simulink model "fp_demo"  (Simulink 6.3)
settings: Solver=FixedStepDiscrete  StartTime=0.0  StopTime=samps+8  RelTol=1e-3
PreLoadFcn:
  | testmult
InitFcn:
  | %% DSPBuilder Start
  | alt_dspbuilder_update_model(bdroot)
  | %% DSPBuilder End
undefined symbols (not defined in the file or in its folder): fplib, FPMULT_HW
libraries: allblocks_alteradspbuilder2 x112
settings Model: Creator=mjervis  LastModifiedBy=LKONG
settings OptimizationCC: InlineInvariantSignals=on
settings DebuggingCC: SolverPrmCheckMsg=none
settings HardwareCC: TargetUnknown=on

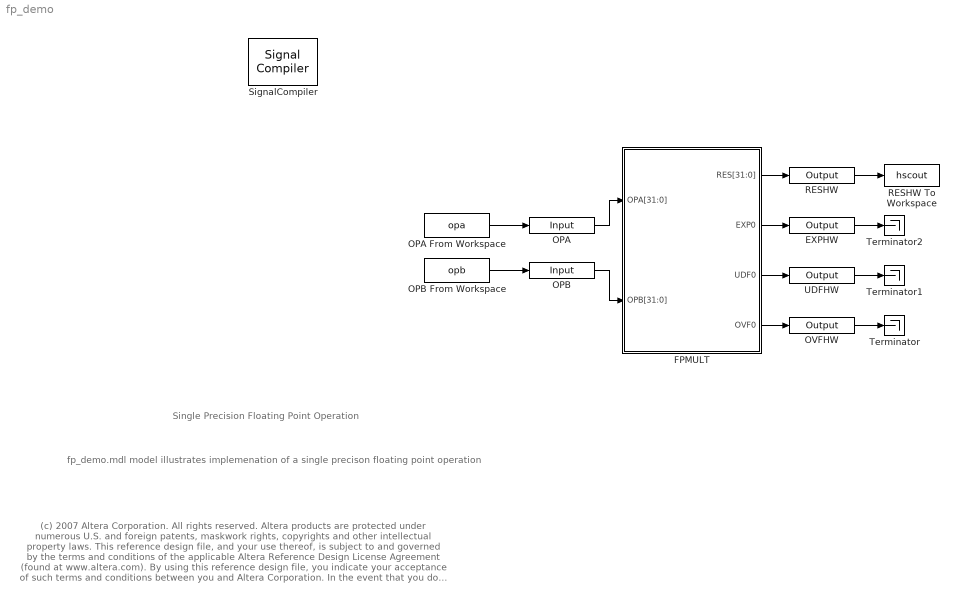
== system fp_demo ==
  note: (c) 2007 Altera Corporation. All rights reserved.  Altera products are protected under numerous U.S. and foreign patents, maskwork rights, copyrights and other intellectual property laws.
      | This reference design file, and your use thereof, is subject to and governed by the terms and conditions of the applicable Altera Reference Design License Agreement (found at www.altera.com).
      | By using this reference design file, you indicate your acceptance of such terms and conditions between you and Altera Corporation.
      | In the event that you do not agree with such terms and conditions, you may not use the reference design file and please promptly destroy any copies you have made.
      | This reference design file being provided on an "as-is" basis and as an accommodation and therefore all warranties, representations or guarantees of any kind (whether express, implied or statutory)
      | including, without limitation, warranties of merchantability, non-infringement, or fitness for a particular purpose, are specifically disclaimed.
      | By making this reference design file available, Altera expressly does not recommend, suggest or require that this reference design file be used in combination with any other product not provided by Altera
  note: Single Precision Floating Point Operation
  note: fp_demo.mdl model illustrates implemenation of a single precison floating point operation
  EXPHW : allblocks_alteradspbuilder2/Output  iofile=d:\wsTrunk\workspace\Documentation\DesignExamples\Demos\fp\Arithm\tb_fp_demo\fp_demo_EXPHW.capture  BusType=Single Bit  bwl=1  bwr=0  PORTTYPE=Output
  FPMULT : Subsystem  AncestorBlock=fplib/FPMULT_HW
      mask Type: SubSystem AlteraBlockSet
  OPA : allblocks_alteradspbuilder2/Input  iofile=d:\wsTrunk\workspace\Documentation\DesignExamples\Demos\fp\Arithm\tb_fp_demo\fp_demo_OPA.salt  BusType=Unsigned Integer  bwl=32  bwr=0  SpecifyClock=off  PORTTYPE=Input
  OPA From Workspace : FromWorkspace  VariableName=opa  SampleTime=1  Interpolate=off  OutputAfterFinalValue=Setting to zero
  OPB : allblocks_alteradspbuilder2/Input  iofile=d:\wsTrunk\workspace\Documentation\DesignExamples\Demos\fp\Arithm\tb_fp_demo\fp_demo_OPB.salt  BusType=Unsigned Integer  bwl=32  bwr=0  SpecifyClock=off  PORTTYPE=Input
  OPB From Workspace : FromWorkspace  VariableName=opb  SampleTime=1  Interpolate=off  OutputAfterFinalValue=Setting to zero
  OVFHW : allblocks_alteradspbuilder2/Output  iofile=d:\wsTrunk\workspace\Documentation\DesignExamples\Demos\fp\Arithm\tb_fp_demo\fp_demo_OVFHW.capture  BusType=Single Bit  bwl=1  bwr=0  PORTTYPE=Output
  RESHW : allblocks_alteradspbuilder2/Output  iofile=d:\wsTrunk\workspace\Documentation\DesignExamples\Demos\fp\Arithm\tb_fp_demo\fp_demo_RESHW.capture  BusType=Unsigned Integer  bwl=32  bwr=0  PORTTYPE=Output
  RESHW To Workspace : ToWorkspace  VariableName=hscout  SampleTime=-1  SaveFormat=Array
  SignalCompiler : allblocks_alteradspbuilder2/Signal Compiler  DeviceFamily=Stratix III  DeviceName=AUTO  EnableSignalTap=off  SignalTapDepth=128  UseBoardBlock=off  StpUseDefaultClock=on  StpClock=clock
  Terminator : Terminator
  Terminator1 : Terminator
  Terminator2 : Terminator
  UDFHW : allblocks_alteradspbuilder2/Output  iofile=d:\wsTrunk\workspace\Documentation\DesignExamples\Demos\fp\Arithm\tb_fp_demo\fp_demo_UDFHW.capture  BusType=Single Bit  bwl=1  bwr=0  PORTTYPE=Output
  wires:
  FPMULT/1(RES[31:0]) -> RESHW/1
  FPMULT/2(EXP0) -> EXPHW/1
  FPMULT/3(UDF0) -> UDFHW/1
  FPMULT/4(OVF0) -> OVFHW/1
  RESHW/1 -> RESHW To Workspace/1
  OPA From Workspace/1 -> OPA/1
  OPB From Workspace/1 -> OPB/1
  OPB/1 -> FPMULT/2(OPB[31:0])
  OPA/1 -> FPMULT/1(OPA[31:0])
  OVFHW/1 -> Terminator/1
  EXPHW/1 -> Terminator2/1
  UDFHW/1 -> Terminator1/1

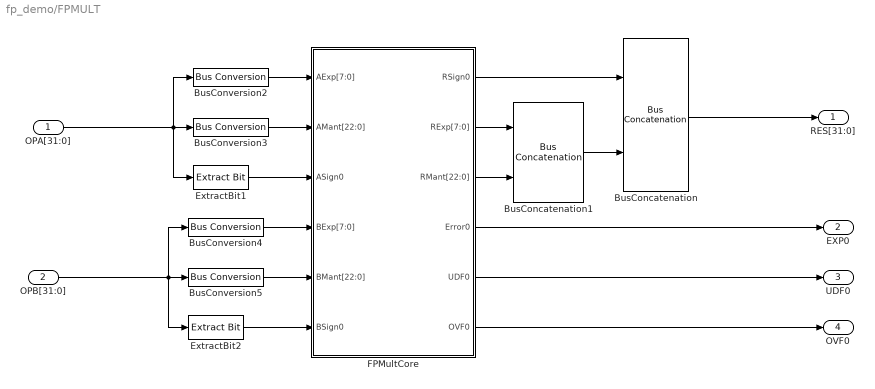
== system fp_demo/FPMULT ==
  OPA[31:0] : Inport
  OPB[31:0] : Inport  Port=2
  BusConcatenation : allblocks_alteradspbuilder2/Bus Concatenation  isSigned=off  awidth=1  bwidth=31
  BusConcatenation1 : allblocks_alteradspbuilder2/Bus Concatenation  isSigned=off  awidth=8  bwidth=23
  BusConversion2 : allblocks_alteradspbuilder2/Bus Conversion  BusType=Unsigned Integer  ibwl=32  ibwr=0  bwl=8  bwr=0  bitToConnectToOutputLSB=23  round=off  saturate=off
  BusConversion3 : allblocks_alteradspbuilder2/Bus Conversion  BusType=Unsigned Integer  ibwl=32  ibwr=0  bwl=23  bwr=0  bitToConnectToOutputLSB=0  round=off  saturate=off
  BusConversion4 : allblocks_alteradspbuilder2/Bus Conversion  BusType=Unsigned Integer  ibwl=32  ibwr=0  bwl=8  bwr=0  bitToConnectToOutputLSB=23  round=off  saturate=off
  BusConversion5 : allblocks_alteradspbuilder2/Bus Conversion  BusType=Unsigned Integer  ibwl=32  ibwr=0  bwl=23  bwr=0  bitToConnectToOutputLSB=0  round=off  saturate=off
  ExtractBit1 : allblocks_alteradspbuilder2/Extract Bit  BusType=Signed Fractional  bwl=32  bwr=0  bitToSelect=31
  ExtractBit2 : allblocks_alteradspbuilder2/Extract Bit  BusType=Signed Fractional  bwl=32  bwr=0  bitToSelect=31
  FPMultCore : Subsystem  AncestorBlock=ALTELINK/AltLab/HDL SubSystem
      mask Type: SubSystem AlteraBlockSet
  RES[31:0] : Outport
  EXP0 : Outport  Port=2
  UDF0 : Outport  Port=3
  OVF0 : Outport  Port=4
  wires:
  FPMultCore/6(OVF0) -> OVF0/1
  FPMultCore/5(UDF0) -> UDF0/1
  FPMultCore/4(Error0) -> EXP0/1
  BusConcatenation/1 -> RES[31:0]/1
  BusConcatenation1/1 -> BusConcatenation/2
  FPMultCore/2(RExp[7:0]) -> BusConcatenation1/1
  FPMultCore/3(RMant[22:0]) -> BusConcatenation1/2
  FPMultCore/1(RSign0) -> BusConcatenation/1
  ExtractBit2/1 -> FPMultCore/6(BSign0)
  BusConversion5/1 -> FPMultCore/5(BMant[22:0])
  BusConversion4/1 -> FPMultCore/4(BExp[7:0])
  ExtractBit1/1 -> FPMultCore/3(ASign0)
  BusConversion3/1 -> FPMultCore/2(AMant[22:0])
  BusConversion2/1 -> FPMultCore/1(AExp[7:0])
  OPA[31:0]/1 -> ExtractBit1/1, BusConversion3/1, BusConversion2/1
  OPB[31:0]/1 -> BusConversion4/1, BusConversion5/1, ExtractBit2/1

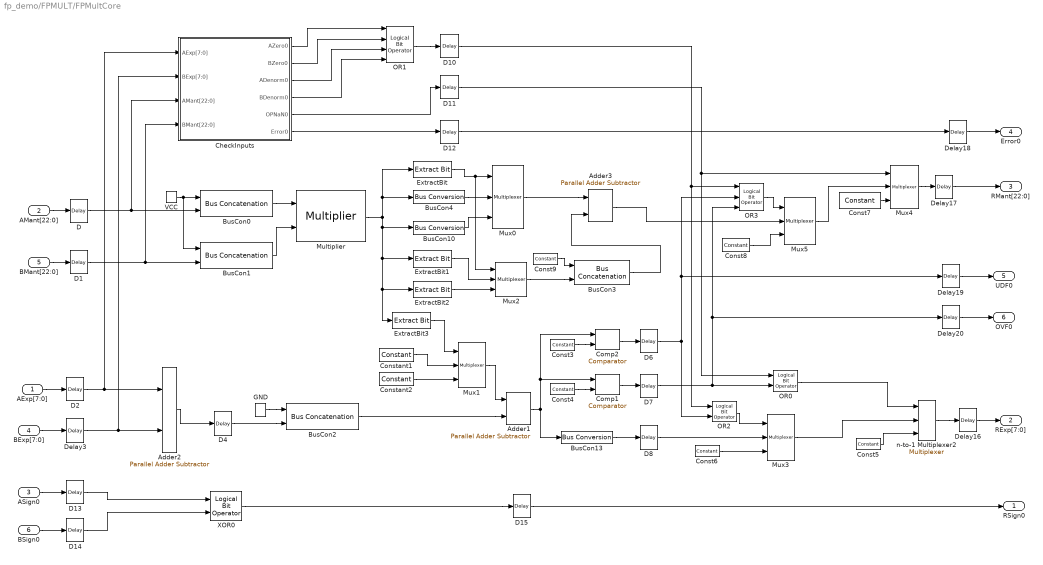
== system fp_demo/FPMULT/FPMultCore ==
  AExp[7:0] : Inport
  AMant[22:0] : Inport  Port=2
  ASign0 : Inport  Port=3
  BExp[7:0] : Inport  Port=4
  BMant[22:0] : Inport  Port=5
  BSign0 : Inport  Port=6
  Adder1 : allblocks_alteradspbuilder2/Parallel Adder Subtractor  number_of_inputs=2  direction=-+  use_pipeline=on  phase_selection=1  use_ena=off  use_aclr=off
  Adder2 : allblocks_alteradspbuilder2/Parallel Adder Subtractor  number_of_inputs=2  direction=++  use_pipeline=on  phase_selection=1  use_ena=off  use_aclr=off
  Adder3 : allblocks_alteradspbuilder2/Parallel Adder Subtractor  number_of_inputs=2  direction=++  use_pipeline=on  phase_selection=1  use_ena=off  use_aclr=off
  BusCon0 : allblocks_alteradspbuilder2/Bus Concatenation  isSigned=off  awidth=1  bwidth=23
  BusCon1 : allblocks_alteradspbuilder2/Bus Concatenation  isSigned=off  awidth=1  bwidth=23
  BusCon10 : allblocks_alteradspbuilder2/Bus Conversion  BusType=Unsigned Integer  ibwl=48  ibwr=0  bwl=23  bwr=0  bitToConnectToOutputLSB=24  round=off  saturate=off
  BusCon13 : allblocks_alteradspbuilder2/Bus Conversion  BusType=Unsigned Integer  ibwl=11  ibwr=0  bwl=8  bwr=0  bitToConnectToOutputLSB=0  round=on  saturate=on
  BusCon2 : allblocks_alteradspbuilder2/Bus Concatenation  isSigned=on  awidth=1  bwidth=9
  BusCon3 : allblocks_alteradspbuilder2/Bus Concatenation  isSigned=off  awidth=22  bwidth=1
  BusCon4 : allblocks_alteradspbuilder2/Bus Conversion  BusType=Unsigned Integer  ibwl=48  ibwr=0  bwl=23  bwr=0  bitToConnectToOutputLSB=23  round=off  saturate=off
  CheckInputs : Subsystem  AncestorBlock=ALTELINK/AltLab/HDL SubSystem
      mask Type: SubSystem AlteraBlockSet
  Comp1 : allblocks_alteradspbuilder2/Comparator  direction=a >= b
  Comp2 : allblocks_alteradspbuilder2/Comparator  direction=a <= b
  Const3 : allblocks_alteradspbuilder2/Constant  mask_cst=0  BusType=Signed Integer  bwl=11  bwr=0  SpecifyClock=off
  Const4 : allblocks_alteradspbuilder2/Constant  mask_cst=255  BusType=Signed Integer  bwl=11  bwr=0  SpecifyClock=off
  Const5 : allblocks_alteradspbuilder2/Constant  mask_cst=255  BusType=Unsigned Integer  bwl=8  bwr=0  SpecifyClock=off
  Const6 : allblocks_alteradspbuilder2/Constant  mask_cst=0  BusType=Unsigned Integer  bwl=8  bwr=0  SpecifyClock=off
  Const7 : allblocks_alteradspbuilder2/Constant  mask_cst=(2^23)-1  BusType=Unsigned Integer  bwl=23  bwr=0  SpecifyClock=off
  Const8 : allblocks_alteradspbuilder2/Constant  mask_cst=0  BusType=Unsigned Integer  bwl=23  bwr=0  SpecifyClock=off
  Const9 : allblocks_alteradspbuilder2/Constant  mask_cst=0  BusType=Unsigned Integer  bwl=22  bwr=0  SpecifyClock=off
  Constant1 : allblocks_alteradspbuilder2/Constant  mask_cst=127  BusType=Signed Integer  bwl=10  bwr=0  SpecifyClock=off
  Constant2 : allblocks_alteradspbuilder2/Constant  mask_cst=126  BusType=Signed Integer  bwl=10  bwr=0  SpecifyClock=off
  D{,1..2,6..8,13..14} (8 alike) : allblocks_alteradspbuilder2/Delay  pipeline=1  ClockPhase=1  use_ena=off  use_sclr=off  use_init=off  reset_value=1
  D10 : allblocks_alteradspbuilder2/Delay  pipeline=4  ClockPhase=1  use_ena=off  use_sclr=off  use_init=off  reset_value=1
  D11 : allblocks_alteradspbuilder2/Delay  pipeline=4  ClockPhase=1  use_ena=off  use_sclr=off  use_init=off  reset_value=1
  D12 : allblocks_alteradspbuilder2/Delay  pipeline=5  ClockPhase=1  use_ena=off  use_sclr=off  use_init=off  reset_value=1
  D15 : allblocks_alteradspbuilder2/Delay  pipeline=6  ClockPhase=1  use_ena=off  use_sclr=off  use_init=off  reset_value=1
  D4 : allblocks_alteradspbuilder2/Delay  pipeline=2  ClockPhase=1  use_ena=off  use_sclr=off  use_init=off  reset_value=1
  Delay{3,16..20} (6 alike) : allblocks_alteradspbuilder2/Delay  pipeline=1  ClockPhase=1  use_ena=off  use_sclr=off  use_init=off  reset_value=1
  ExtractBit : allblocks_alteradspbuilder2/Extract Bit  BusType=Signed Fractional  bwl=48  bwr=0  bitToSelect=47
  ExtractBit1 : allblocks_alteradspbuilder2/Extract Bit  BusType=Signed Fractional  bwl=48  bwr=0  bitToSelect=22
  ExtractBit2 : allblocks_alteradspbuilder2/Extract Bit  BusType=Signed Fractional  bwl=48  bwr=0  bitToSelect=23
  ExtractBit3 : allblocks_alteradspbuilder2/Extract Bit  BusType=Signed Fractional  bwl=48  bwr=0  bitToSelect=47
  GND : allblocks_alteradspbuilder2/GND  SpecifyClock=off
  Multiplier : allblocks_alteradspbuilder2/Multiplier  BusType=Unsigned Integer  bwl=24  bwr=0  pipeline=3  UseEqualInputWidth=on  bbwl=24  bbwr=0  FullResolution=on  OutputMsb=47  OutputLsb=0  OutputBwl=48  OutputBwr=0  UseDedicatedCircuitry=AUTO  use_ena=off  use_aclr=off
  Mux0 : allblocks_alteradspbuilder2/Multiplexer  numInputs=2  pipeline=1  oneHot=off  use_ena=off  use_aclr=off
  Mux{1,3..5} (4 alike) : allblocks_alteradspbuilder2/Multiplexer  numInputs=2  pipeline=0  oneHot=off  use_ena=off  use_aclr=off
  Mux2 : allblocks_alteradspbuilder2/Multiplexer  numInputs=2  pipeline=1  oneHot=off  use_ena=off  use_aclr=off
  OR0 : allblocks_alteradspbuilder2/Logical Bit Operator  LogicalOperator=OR  user_inputs=2
  OR1 : allblocks_alteradspbuilder2/Logical Bit Operator  LogicalOperator=OR  user_inputs=4
  OR2 : allblocks_alteradspbuilder2/Logical Bit Operator  LogicalOperator=OR  user_inputs=2
  OR3 : allblocks_alteradspbuilder2/Logical Bit Operator  LogicalOperator=OR  user_inputs=3
  VCC : allblocks_alteradspbuilder2/VCC  SpecifyClock=off
  XOR0 : allblocks_alteradspbuilder2/Logical Bit Operator  LogicalOperator=XOR  user_inputs=2
  n-to-1 Multiplexer2 : allblocks_alteradspbuilder2/Multiplexer  numInputs=2  pipeline=0  oneHot=off  use_ena=off  use_aclr=off
  RSign0 : Outport
  RExp[7:0] : Outport  Port=2
  RMant[22:0] : Outport  Port=3
  Error0 : Outport  Port=4
  UDF0 : Outport  Port=5
  OVF0 : Outport  Port=6
  wires:
  Const8/1 -> Mux5/3
  OR3/1 -> Mux5/1
  CheckInputs/1(AZero0) -> OR1/1
  ExtractBit3/1 -> Mux1/1
  D2/1 -> CheckInputs/1(AExp[7:0]), Adder2/1
  Delay3/1 -> CheckInputs/2(BExp[7:0]), Adder2/2
  Const9/1 -> BusCon3/1
  Mux2/1 -> BusCon3/2
  BusCon3/1 -> Adder3/2
  ExtractBit1/1 -> Mux2/2
  ExtractBit2/1 -> Mux2/3
  Adder3/1 -> Mux5/2
  Mux0/1 -> Adder3/1
  Delay20/1 -> OVF0/1
  Delay19/1 -> UDF0/1
  Delay18/1 -> Error0/1
  D12/1 -> Delay18/1
  Delay17/1 -> RMant[22:0]/1
  Delay16/1 -> RExp[7:0]/1
  Mux4/1 -> Delay17/1
  n-to-1 Multiplexer2/1 -> Delay16/1
  XOR0/1 -> D15/1
  D14/1 -> XOR0/2
  D13/1 -> XOR0/1
  BSign0/1 -> D14/1
  ASign0/1 -> D13/1
  Mux5/1 -> Mux4/2
  Const7/1 -> Mux4/3
  D10/1 -> OR3/1, OR2/1
  D8/1 -> Mux3/2
  D6/1 -> OR2/2, OR3/2, Delay19/1
  OR2/1 -> Mux3/1
  Const6/1 -> Mux3/3
  Mux3/1 -> n-to-1 Multiplexer2/2
  Const5/1 -> n-to-1 Multiplexer2/3
  D11/1 -> OR0/1, Mux4/1
  D7/1 -> Delay20/1, OR3/3, OR0/2
  OR1/1 -> D10/1
  OR0/1 -> n-to-1 Multiplexer2/1
  CheckInputs/6(Error0) -> D12/1
  CheckInputs/5(OPNaN0) -> D11/1
  CheckInputs/4(BDenorm0) -> OR1/4
  CheckInputs/3(ADenorm0) -> OR1/3
  CheckInputs/2(BZero0) -> OR1/2
  BusCon13/1 -> D8/1
  Comp1/1 -> D7/1
  Comp2/1 -> D6/1
  Const4/1 -> Comp1/2
  Const3/1 -> Comp2/2
  Adder1/1 -> Comp1/1, Comp2/1, BusCon13/1
  GND/1 -> BusCon2/1
  BusCon2/1 -> Adder1/2
  Mux1/1 -> Adder1/1
  Constant2/1 -> Mux1/3
  Constant1/1 -> Mux1/2
  D4/1 -> BusCon2/2
  Adder2/1 -> D4/1
  ExtractBit/1 -> Mux2/1, Mux0/1
  BusCon10/1 -> Mux0/3
  BusCon4/1 -> Mux0/2
  VCC/1 -> BusCon0/1, BusCon1/1
  BusCon1/1 -> Multiplier/2
  BusCon0/1 -> Multiplier/1
  BMant[22:0]/1 -> D1/1
  BExp[7:0]/1 -> Delay3/1
  AMant[22:0]/1 -> D/1
  AExp[7:0]/1 -> D2/1
  D/1 -> BusCon0/2, CheckInputs/3(AMant[22:0])
  D1/1 -> BusCon1/2, CheckInputs/4(BMant[22:0])
  Multiplier/1 -> ExtractBit/1, BusCon4/1, BusCon10/1, ExtractBit1/1, ExtractBit3/1, ExtractBit2/1
  D15/1 -> RSign0/1

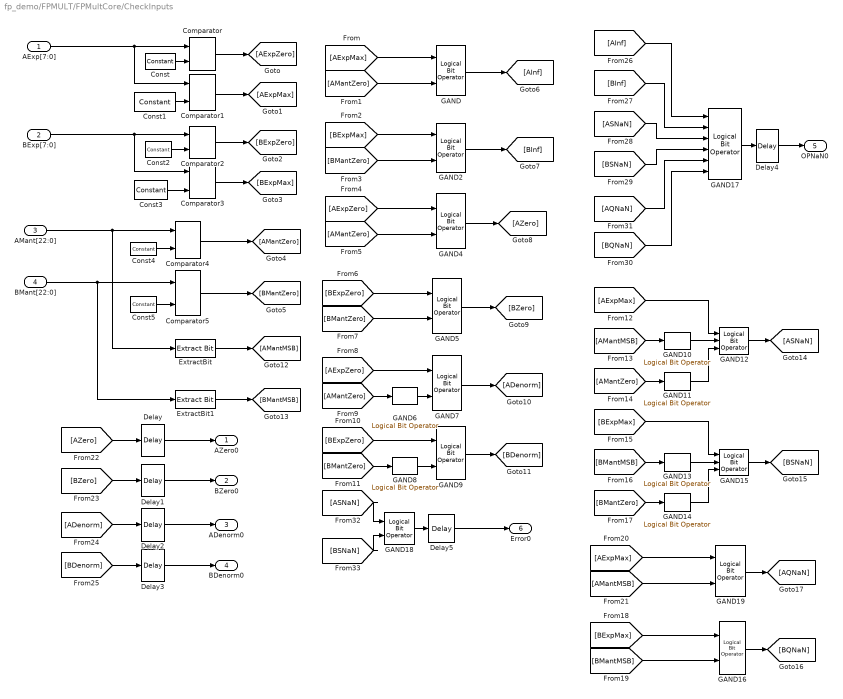
== system fp_demo/FPMULT/FPMultCore/CheckInputs ==
  AExp[7:0] : Inport
  BExp[7:0] : Inport  Port=2
  AMant[22:0] : Inport  Port=3
  BMant[22:0] : Inport  Port=4
  Comparator{,1..5} (6 alike) : allblocks_alteradspbuilder2/Comparator  direction=a == b
  Const : allblocks_alteradspbuilder2/Constant  mask_cst=0  BusType=Unsigned Integer  bwl=8  bwr=0  SpecifyClock=off
  Const1 : allblocks_alteradspbuilder2/Constant  mask_cst=255  BusType=Unsigned Integer  bwl=8  bwr=0  SpecifyClock=off
  Const2 : allblocks_alteradspbuilder2/Constant  mask_cst=0  BusType=Unsigned Integer  bwl=8  bwr=0  SpecifyClock=off
  Const3 : allblocks_alteradspbuilder2/Constant  mask_cst=255  BusType=Unsigned Integer  bwl=8  bwr=0  SpecifyClock=off
  Const4 : allblocks_alteradspbuilder2/Constant  mask_cst=0  BusType=Unsigned Integer  bwl=23  bwr=0  SpecifyClock=off
  Const5 : allblocks_alteradspbuilder2/Constant  mask_cst=0  BusType=Unsigned Integer  bwl=23  bwr=0  SpecifyClock=off
  Delay{,1..5} (6 alike) : allblocks_alteradspbuilder2/Delay  pipeline=1  ClockPhase=1  use_ena=off  use_sclr=off  use_init=off  reset_value=1
  ExtractBit : allblocks_alteradspbuilder2/Extract Bit  BusType=Signed Fractional  bwl=23  bwr=0  bitToSelect=22
  ExtractBit1 : allblocks_alteradspbuilder2/Extract Bit  BusType=Signed Fractional  bwl=23  bwr=0  bitToSelect=22
  GAND{,2,4..5,7,9,16,19} (8 alike) : allblocks_alteradspbuilder2/Logical Bit Operator  LogicalOperator=AND  user_inputs=2
  GAND{6,8,10..11,13..14} (6 alike) : allblocks_alteradspbuilder2/Logical Bit Operator  LogicalOperator=NOT  user_inputs=2
  GAND12 : allblocks_alteradspbuilder2/Logical Bit Operator  LogicalOperator=AND  user_inputs=3
  GAND15 : allblocks_alteradspbuilder2/Logical Bit Operator  LogicalOperator=AND  user_inputs=3
  GAND17 : allblocks_alteradspbuilder2/Logical Bit Operator  LogicalOperator=OR  user_inputs=6
  GAND18 : allblocks_alteradspbuilder2/Logical Bit Operator  LogicalOperator=OR  user_inputs=2
  AZero0 : Outport
  BZero0 : Outport  Port=2
  ADenorm0 : Outport  Port=3
  BDenorm0 : Outport  Port=4
  OPNaN0 : Outport  Port=5
  Error0 : Outport  Port=6
  wires:
  BMant[22:0]/1 -> ExtractBit1/1, Comparator5/1
  AMant[22:0]/1 -> ExtractBit/1, Comparator4/1
  BExp[7:0]/1 -> Comparator3/1, Comparator2/1
  AExp[7:0]/1 -> Comparator/1, Comparator1/1
  Delay4/1 -> OPNaN0/1
  Delay3/1 -> BDenorm0/1
  Delay2/1 -> ADenorm0/1
  Delay1/1 -> BZero0/1
  Delay/1 -> AZero0/1
  GAND18/1 -> Delay5/1
  [BSNaN] -> GAND18/2
  [ASNaN] -> GAND18/1
  [BQNaN] -> GAND17/6
  [AQNaN] -> GAND17/5
  [BSNaN] -> GAND17/4
  [ASNaN] -> GAND17/3
  [BInf] -> GAND17/2
  [AInf] -> GAND17/1
  GAND17/1 -> Delay4/1
  [BDenorm] -> Delay3/1
  [ADenorm] -> Delay2/1
  [BZero] -> Delay1/1
  [AZero] -> Delay/1
  GAND16/1 -> [BQNaN]
  [BExpMax] -> GAND16/1
  [BMantMSB] -> GAND16/2
  GAND19/1 -> [AQNaN]
  [AExpMax] -> GAND19/1
  [AMantMSB] -> GAND19/2
  GAND15/1 -> [BSNaN]
  GAND14/1 -> GAND15/3
  GAND13/1 -> GAND15/2
  [BExpMax] -> GAND15/1
  [BMantZero] -> GAND14/1
  [BMantMSB] -> GAND13/1
  GAND12/1 -> [ASNaN]
  GAND11/1 -> GAND12/3
  GAND10/1 -> GAND12/2
  [AExpMax] -> GAND12/1
  [AMantZero] -> GAND11/1
  [AMantMSB] -> GAND10/1
  ExtractBit1/1 -> [BMantMSB]
  ExtractBit/1 -> [AMantMSB]
  GAND9/1 -> [BDenorm]
  GAND8/1 -> GAND9/2
  [BMantZero] -> GAND8/1
  [BExpZero] -> GAND9/1
  GAND7/1 -> [ADenorm]
  GAND6/1 -> GAND7/2
  [AMantZero] -> GAND6/1
  [AExpZero] -> GAND7/1
  GAND5/1 -> [BZero]
  [BMantZero] -> GAND5/2
  [BExpZero] -> GAND5/1
  GAND4/1 -> [AZero]
  [AMantZero] -> GAND4/2
  [AExpZero] -> GAND4/1
  GAND2/1 -> [BInf]
  GAND/1 -> [AInf]
  [BMantZero] -> GAND2/2
  [BExpMax] -> GAND2/1
  [AMantZero] -> GAND/2
  [AExpMax] -> GAND/1
  Comparator5/1 -> [BMantZero]
  Comparator4/1 -> [AMantZero]
  Const5/1 -> Comparator5/2
  Const4/1 -> Comparator4/2
  Comparator3/1 -> [BExpMax]
  Comparator2/1 -> [BExpZero]
  Const3/1 -> Comparator3/2
  Const2/1 -> Comparator2/2
  Comparator1/1 -> [AExpMax]
  Comparator/1 -> [AExpZero]
  Const1/1 -> Comparator1/2
  Const/1 -> Comparator/2
  Delay5/1 -> Error0/1
